simulink subsystem "tehrani_tissue_mass_balance_v2"  (R2019b)
settings: Solver=VariableStepAuto  StartTime=0.0  StopTime=10.0  RelTol=1e-3
settings Model: Creator=RH  LastModifiedBy=RH

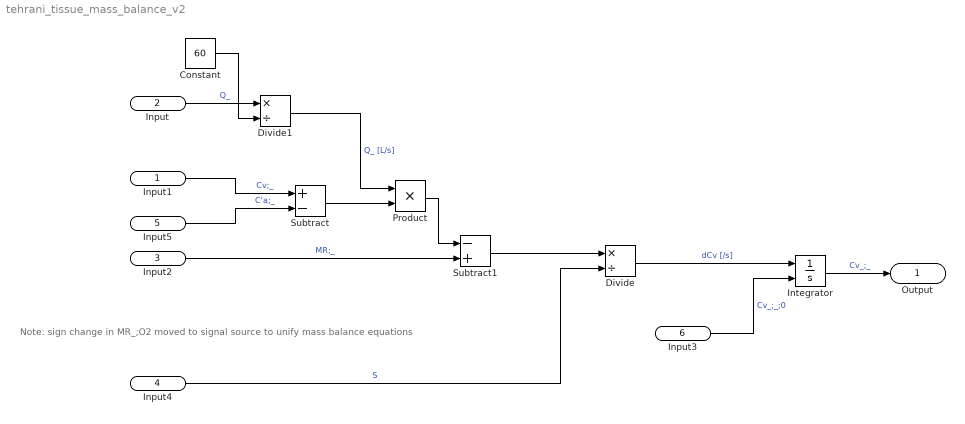
== system tehrani_tissue_mass_balance_v2 ==
  note: Note: sign change in MR_;O2 moved to signal source to unify mass balance equations
  Input1 : Inport  Unit=1
  Input : Inport  Port=2  Unit=liter/minute
  Input2 : Inport  Port=3  Unit=liter/second
  Input4 : Inport  Port=4  Unit=liter
  Input5 : Inport  Port=5  Unit=1
  Input3 : Inport  Port=6  Unit=1
  Constant : Constant  Value=60
  Divide : Product  Inputs=*/
  Divide1 : Product  Inputs=*/
  Integrator : Integrator  InitialConditionSource=external
  Product : Product
  Subtract : Sum  Inputs=+-
  Subtract1 : Sum  Inputs=-+
  Output : Outport  Unit=1
  wires:
  Input3/1 -> Integrator/2  "Cv_;_;0"
  Constant/1 -> Divide1/2
  Input1/1 -> Subtract/1  "Cv;_"
  Input5/1 -> Subtract/2  "C'a;_"
  Subtract/1 -> Product/2
  Input/1 -> Divide1/1  "Q_"
  Product/1 -> Subtract1/1
  Input2/1 -> Subtract1/2  "MR;_"
  Subtract1/1 -> Divide/1
  Input4/1 -> Divide/2  "S"
  Divide/1 -> Integrator/1  "dCv [/s]"
  Divide1/1 -> Product/1  "Q_ [L/s]"
  Integrator/1 -> Output/1  "Cv_;_"
